simulink library "lib_brake_torque_cal_nodiv"  (Simulink 7.7)
settings: Solver=ode45  SolverMode=SingleTasking  StartTime=0.0  StopTime=10.0  RelTol=1e-3
PreLoadFcn:
  | if exist('tl_preloadfcn','file'), tl_preloadfcn(gcs,101); end
PostLoadFcn:
  | if exist('tl_postloadfcn','file'), tl_postloadfcn(gcs,101); end
undefined symbols (not defined in the file): maxBrakeTorque
settings Model: TLRevision=101  Creator=yt59680  LastModifiedBy=lfeng

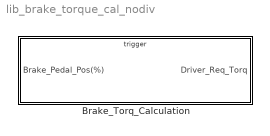
== system lib_brake_torque_cal_nodiv ==
  Brake_Torq_Calculation : Subsystem  TreatAsAtomicUnit=on

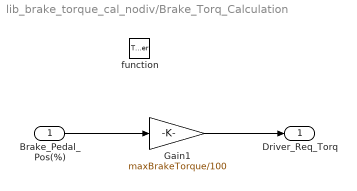
== system lib_brake_torque_cal_nodiv/Brake_Torq_Calculation ==
  Brake_Pedal_Pos(%) : Inport
  function : TriggerPort  TriggerType=function-call
  Gain1 : Gain  Gain=maxBrakeTorque/100  OutMin=0  OutMax=4000
  Driver_Req_Torq : Outport
  wires:
  Brake_Pedal_Pos(%)/1 -> Gain1/1
  Gain1/1 -> Driver_Req_Torq/1
